simulink model "PMSMSystem"  (R2025a)
settings: Solver=ode45  StartTime=0.0  StopTime=0.2  FixedStep=40e-6  RelTol=1e-3
PreLoadFcn:
  | pmsmfoc_data
StartFcn:
  | clear executionProfile
StopFcn:
  | try
  |   AddExecutionProfileToDataInspector();
  | end
undefined symbols (not defined in the file): ctrlConst, DiscIntNeverNeededParam, EnumCommandType, pmsm, sensors
libraries: fl_lib x13, nesl_utility x11, ee_lib x6, fl_ps_legacy_lib x2, simulink x2, eeTransforms x1, SignalEditorBlockLib x1
Description:
  | Field-Oriented Control of Permanent Magnet Synchronous Machine
  | 
  | Demonstrates a Field-Oriented Control algorithm with Space Vector Modulation for a Permanent Magnet Synchronous Machine (PMSM).
  | The test bench can be used to evaluate the system performance. Examples include turning the motor on, searching for a valid rotor position,
  | transitioning to closed loop operation, and changing speed and torque during closed loop control.
  | The Embedded Processor subsystem contains the controller algorithm (which supports C code generation) as well as simulation models of peripherals.
settings Model: Creator=The MathWorks, Inc.  LastModifiedBy=anubhasinghal
settings SolverCC: AlgebraicLoopSolver=TrustRegion
settings DataIOCC: LimitDataPoints=on  SaveFormat=Array  SaveOutput=off  SaveTime=off
settings OptimizationCC: DefaultParameterBehavior=Inlined  UseFloatMulNetSlope=on  InlineInvariantSignals=on  ReuseModelBlockBuffer=off  EnhancedBackFolding=on  StrengthReduction=on  PassReuseOutputArgsAs=Individual arguments  ExpressionDepthLimit=2147483647.0  ZeroExternalMemoryAtStartup=off  EfficientFloat2IntCast=on  LifeSpan=1  EfficientTunableParamExpr=on
settings DebuggingCC: AlgebraicLoopMsg=error  MergeDetectMultiDrivingBlocksExec=none  SingleTaskRateTransMsg=error  IntegerOverflowMsg=none  ParameterPrecisionLossMsg=none  FcnCallInpInsideContextMsg=warning  UniqueDataStoreMsg=error  AssertControl=DisableAll  AllowSymbolicDim=off  StateNameClashWarn=warning  SubsystemReferenceDiagnosticForUnitTest=warning  SFUnexpectedBacktrackingDiag=warning  SFNoUnconditionalDefaultTransitionDiag=warning  SFExecutionAtInitializationDiag=none  IntegerSaturationMsg=none  ArithmeticOperatorsInVariantConditions=warning
settings ModelReferenceCC: EnableRefExpFcnMdlSchedulingChecks=on  ModelReferenceNumInstancesAllowed=Single  PropagateSignalLabelsOutOfModel=off
settings SFSimCC: SimUseLocalCustomCode=off  MATLABDynamicMemAlloc=off
settings RTWCC: SystemTargetFile=ert.tlc  GenerateMakefile=off  TemplateMakefile=ec_target.tmf  GenerateReport=on  RTWVerbose=off  RTWUseLocalCustomCode=off  IncludeHyperlinkInReport=on  PortableWordSizes=on  CodeExecutionProfiling=on  CodeProfilingSaveOptions=AllData  CodeProfilingInstrumentation=detailed  GenerateTraceInfo=on  GenerateTraceReport=on  GenerateTraceReportSl=on  GenerateTraceReportSf=on  GenerateTraceReportEml=on  GPUComputeCapability=3.5  Description=Embedded Coder
settings CodeAppCC: IgnoreCustomStorageClasses=off  IgnoreTestpoints=on  MaxIdLength=64.0  MATLABFcnDesc=on  CustomSymbolStrGlobalVar=$N$M  CustomSymbolStrType=$N$M  CustomSymbolStrFcn=$N$M$F  CustomSymbolStrFcnArg=$I$N$M  CustomSymbolStrBlkIO=$N$M  CustomSymbolStrMacro=$N$M  StateflowObjectComments=on  MATLABSourceComments=on  InternalIdentifier=Classic
settings ERTTargetCC: ExtModeTransport=0.0  ExtModeStaticAlloc=off  ExtModeMexFile=ext_comm  ExtModeIntrfLevel=Level1  ERTCustomFileTemplate=example_file_process.tlc  ERTFilePackagingFormat=Compact  ConvertIfToSwitch=off  SuppressUnreachableDefaultCases=off  DynamicArrayContainerType=coder::array  MultiwordLength=2048.0  SuppressErrorStatus=on  SupportAbsoluteTime=off  SubcomponentCodeInterfacePackaging=Nonreusable function  SupportNonFinite=off  RemoveResetFunc=off  ParenthesesLevel=Maximum
settings ConfigComp: CovMetricSettings=dcmtrzow  CovHTMLOptions=-aTS=1 -bRG=1 -bTC=1 -hTR=0 -nFC=0 -scm=1 -bcm=1 -xEv=0  CovSaveCumulativeToWorkspaceVar=on  CovSaveSingleToWorkspaceVar=on  CovExternalEMLEnable=off  CovSFcnEnable=off
settings SimscapeCC: SimscapeNormalizeSystem=off

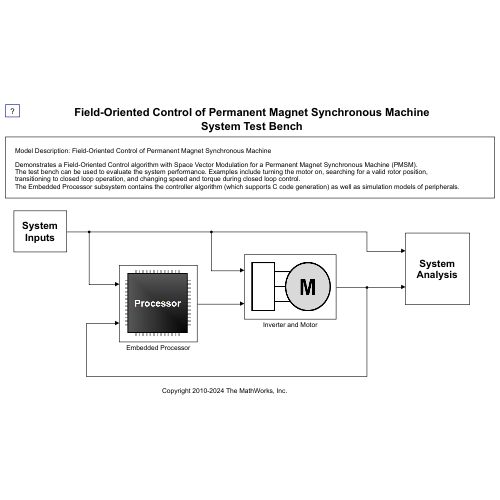
[thumbnail: Simulink's stored preview of the top-level diagram]
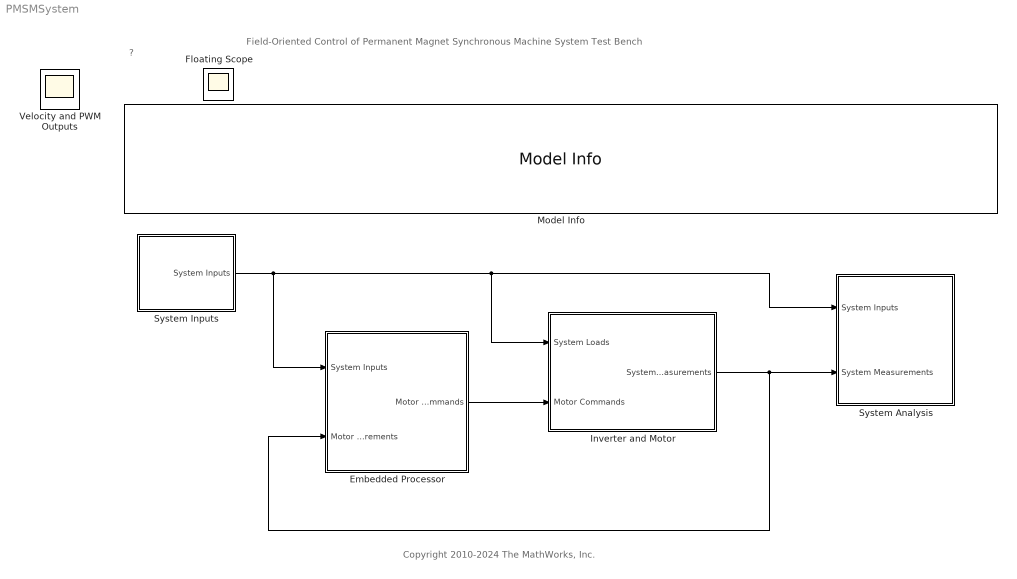
== system PMSMSystem ==
  note: Field-Oriented Control of Permanent Magnet Synchronous Machine
      | System Test Bench
  note: Copyright 2010-2024 The MathWorks, Inc.
  note: ?
  Embedded Processor : Subsystem
      mask Display:
      | if exist('rtwdemo_pmsmfoc_processor.png', 'file')
      |     image('rtwdemo_pmsmfoc_processor.png');
      | end
  Inverter and Motor : Subsystem  Description=""
      mask Display:
      | if exist('rtwdemo_pmsmfoc_motor.png', 'file')
      |     image('rtwdemo_pmsmfoc_motor.png')
      | end
  Model Info : simulink/Model-Wide Utilities/Model Info  Frame=on  DisplayStringWithTags=Model Description: %<Description>  HorizontalTextAlignment=Left  LeftAlignmentValue=0.02
  System Analysis : Subsystem  Description=|
      | System Analysis for Speed Control Design
      | 
      | Analyize and plot signals used to analyize performance of
      | speed  control designs
      mask Display: fprintf('System\nAnalysis')
  System Inputs : Subsystem  Description=""
      mask Display: fprintf('System\nInputs')
  Floating Scope : Scope
  Velocity and PWM Outputs : Scope
      settings: TimeSpan=0.14  ActiveDisplayYMinimum=-500  ActiveDisplayYMaximum=4000  DataLoggingMaxPoints=7500  DataLoggingVariableName=ScopeData4  DataLoggingSaveFormat=Array
  wires:
  Embedded Processor/1(Motor Commands) -> Inverter and Motor/2(Motor Commands)
  Inverter and Motor/1(System Measurements) -> System Analysis/2(System Measurements), Embedded Processor/2(Motor Measurements)
  System Inputs/1(System Inputs) -> System Analysis/1(System Inputs), Inverter and Motor/1(System Loads), Embedded Processor/1(System Inputs)

== system PMSMSystem/Embedded Processor ==
  note: Models hardware on the embedded processor, including
      | the controller algorithm software specification and peripherals.
  note: Embedded Processor
  System Inputs : Inport
  Motor Measurements : Inport  Port=2
  Command Channel : Subsystem  Description=""
      mask Display: fprintf('Command\nChannel')
  Controller Algorithm Software Specification : ModelReference  ModelNameDialog=PMSMController  SimulationMode=Normal  ModelReferenceVersion=11.1
  Driver Peripherals : Subsystem  Description=""
      mask Display: fprintf('Drivers\nPeripherals')
  Sensor Peripherals : Subsystem  Description=|
      | Elaborate Sensor Models
      | 
      | ADC and QEP and Encoder Models
      mask Display: fprintf('Sensor\nPeripherals')
  Motor Commands : Outport  VectorParamsAs1DForOutWhenUnconnected=off
  wires:
  System Inputs/1 -> Command Channel/1(System Inputs)
  Motor Measurements/1 -> Sensor Peripherals/1(System Measurements)
  Driver Peripherals/1(PWM Duty Cycle) -> Motor Commands/1
  Command Channel/1(motor_on) -> Controller Algorithm Software Specification/1  "motor_on"
  Sensor Peripherals/1(Sensors) -> Controller Algorithm Software Specification/4  "sensors"
  Controller Algorithm Software Specification/1 -> Driver Peripherals/1(pwm_compare)  "pwm_compare"
  Command Channel/2(command_type) -> Controller Algorithm Software Specification/2  "command_type"
  Command Channel/3(command_value) -> Controller Algorithm Software Specification/3  "command_value"
  Controller Algorithm Software Specification/2 -> Driver Peripherals/2(error)  "error"

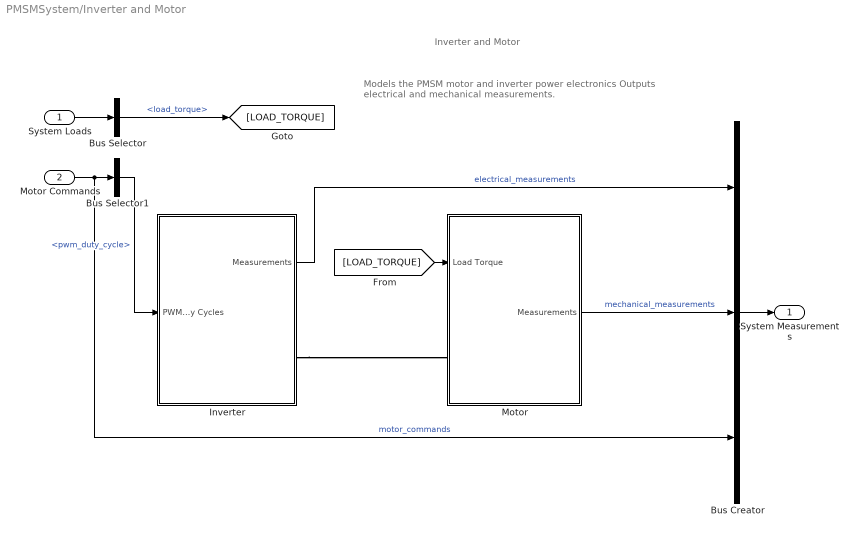
== system PMSMSystem/Inverter and Motor ==
  note: Models the PMSM motor and inverter power electronics
      | Outputs electrical and mechanical measurements.
  note: Inverter and Motor
  System Loads : Inport
  Motor Commands : Inport  Port=2
  Bus Creator : BusCreator  Inputs=3
  Bus Selector : BusSelector  OutputSignals=load_torque
  Bus Selector1 : BusSelector  OutputSignals=pwm_duty_cycle
  Inverter : Subsystem
  Motor : Subsystem
  System Measurements : Outport  VectorParamsAs1DForOutWhenUnconnected=off
  wires:
  Inverter/1(Measurements) -> Bus Creator/1  "electrical_measurements"
  Bus Creator/1 -> System Measurements/1
  Motor/1(Measurements) -> Bus Creator/2  "mechanical_measurements"
  System Loads/1 -> Bus Selector/1
  Motor Commands/1 -> Bus Selector1/1, Bus Creator/3  "motor_commands"
  Bus Selector/1 -> [LOAD_TORQUE]  "<load_torque>"
  Bus Selector1/1 -> Inverter/1(PWM Duty Cycles)  "<pwm_duty_cycle>"
  [LOAD_TORQUE] -> Motor/1("Load Torque ")
  connections:
  Inverter/RConn1 -- Motor/LConn1

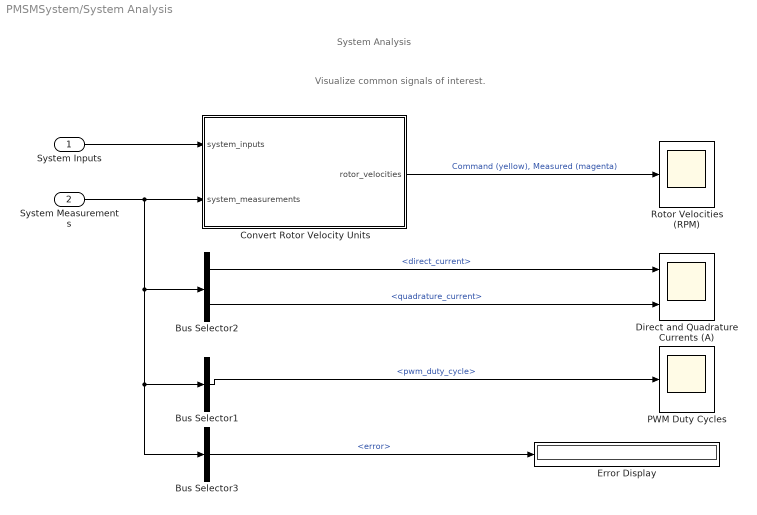
== system PMSMSystem/System Analysis ==
  note: System Analysis
  note: Visualize common signals of interest.
  System Inputs : Inport
  System Measurements : Inport  Port=2
  Bus Selector1 : BusSelector  OutputSignals=motor_commands.pwm_duty_cycle
  Bus Selector2 : BusSelector  OutputSignals=mechanical_measurements.direct_current,mechanical_measurements.quadrature_current
  Bus Selector3 : BusSelector  OutputSignals=motor_commands.error
  Convert Rotor Velocity Units : Subsystem
  Direct and Quadrature Currents (A) : Scope  NumInputPorts=2
      settings: TimeSpan=0.2  ActiveDisplayYMinimum=-0.05574  ActiveDisplayYMaximum=0.11277  DataLoggingVariableName=ScopeData3
  Error Display : Display
  PWM Duty Cycles : Scope
      settings: TimeSpan=1.4  ActiveDisplayYMinimum=0.38629  ActiveDisplayYMaximum=0.61338  DataLoggingVariableName=ScopeData2
  Rotor Velocities (RPM) : Scope
      settings: TimeSpan=0.2  ActiveDisplayYMinimum=-125.00445  ActiveDisplayYMaximum=1125.00049
  wires:
  System Measurements/1 -> Convert Rotor Velocity Units/2(system_measurements), Bus Selector3/1, Bus Selector1/1, Bus Selector2/1
  System Inputs/1 -> Convert Rotor Velocity Units/1(system_inputs)
  Convert Rotor Velocity Units/1(rotor_velocities) -> Rotor Velocities (RPM)/1  "Command (yellow), Measured (magenta)"
  Bus Selector1/1 -> PWM Duty Cycles/1  "<pwm_duty_cycle>"
  Bus Selector2/1 -> Direct and Quadrature Currents (A)/1  "<direct_current>"
  Bus Selector2/2 -> Direct and Quadrature Currents (A)/2  "<quadrature_current>"
  Bus Selector3/1 -> Error Display/1  "<error>"

== system PMSMSystem/System Inputs ==
  note: System Inputs
  note: Specify groups of tests in Signal Builder. Outputs are combined into a bus
      | to simplify signal routing through the model.
  Bus Creator : BusCreator  Inputs=4
  Command Type : simulink/Sources/Enumerated Constant  OutDataTypeStr=Enum: EnumCommandType  Value=EnumCommandType.Velocity  SampleTime=inf
  Signal Editor Experiments : SignalEditorBlockLib/Signal Editor  FileName=rtwdemo_pmsmfoc_system_Signals.mat  ActiveScenario=No_Load_Velocity_Control  ActiveSignal=Load Torque (oz-in)  IsBus=off  OutputBusObjectStr=Bus: BusObject  SampleTime=1e-5  OutputAfterFinalValue=Holding final value  Unit=inherit  PreserveSignalName=on  ApplySigPropsToAllScenarios=on  ApplySigPropsToAllSignals=off  SignalPropertySource=Dialog parameters
  oz-in to Newton Meters : Gain  Gain=0.0070615518333
      settings: AttributesFormatString=-------------------------\n%<Gain>
  rpm to rad per sec : Gain  Gain=pi/30
      settings: AttributesFormatString=------------------\n%<Gain>
  System Inputs : Outport  VectorParamsAs1DForOutWhenUnconnected=off
  wires:
  Bus Creator/1 -> System Inputs/1
  oz-in to Newton Meters/1 -> Bus Creator/4  "load_torque"
  rpm to rad per sec/1 -> Bus Creator/3  "command"
  Command Type/1 -> Bus Creator/1  "command_type"
  Signal Editor Experiments/1 -> Bus Creator/2  "motor_on"
  ? -> rpm to rad per sec/1  "speed_command_rpm"
  ? -> oz-in to Newton Meters/1  "load_torque_ozin"

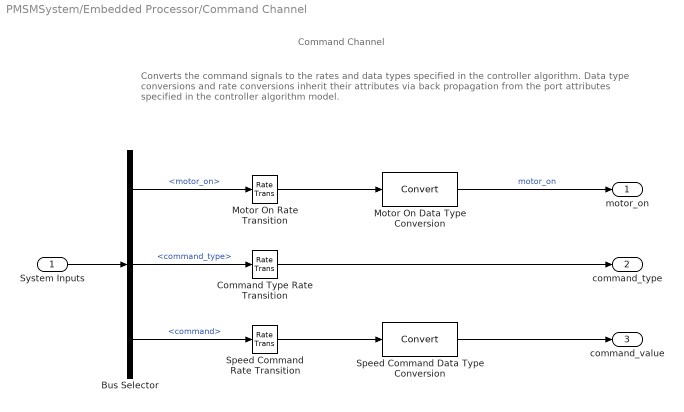
== system PMSMSystem/Embedded Processor/Command Channel ==
  note: Converts the command signals to the rates and data types specified in the controller algorithm.
      | Data type conversions and rate conversions inherit their attributes via back propagation from the
      | port attributes specified in the controller algorithm model.
  note: Command Channel
  System Inputs : Inport
  Bus Selector : BusSelector  OutputSignals=motor_on,command_type,command
  Command Type Rate Transition : RateTransition  Integrity=off  Deterministic=off
  Motor On Data Type Conversion : DataTypeConversion  SaturateOnIntegerOverflow=off  RndMeth=Floor
  Motor On Rate Transition : RateTransition  Integrity=off  Deterministic=off
  Speed Command Data Type Conversion : DataTypeConversion  SaturateOnIntegerOverflow=off  RndMeth=Floor
  Speed Command Rate Transition : RateTransition  Integrity=off  Deterministic=off
  motor_on : Outport  VectorParamsAs1DForOutWhenUnconnected=off
  command_type : Outport  Port=2  VectorParamsAs1DForOutWhenUnconnected=off
  command_value : Outport  Port=3  VectorParamsAs1DForOutWhenUnconnected=off
  wires:
  System Inputs/1 -> Bus Selector/1
  Speed Command Data Type Conversion/1 -> command_value/1
  Bus Selector/1 -> Motor On Rate Transition/1  "<motor_on>"
  Motor On Data Type Conversion/1 -> motor_on/1  "motor_on"
  Motor On Rate Transition/1 -> Motor On Data Type Conversion/1
  Speed Command Rate Transition/1 -> Speed Command Data Type Conversion/1
  Bus Selector/3 -> Speed Command Rate Transition/1  "<command>"
  Bus Selector/2 -> Command Type Rate Transition/1  "<command_type>"
  Command Type Rate Transition/1 -> command_type/1

== system PMSMSystem/Embedded Processor/Driver Peripherals ==
  note: Converts PWM count compare values to a normalized duty cycle.
  note: Driver Peripherals
  pwm_compare : Inport
  error : Inport  Port=2
  Bus Creator : BusCreator  Inputs=2
  Rate Transition : RateTransition  Integrity=off  Deterministic=off  OutPortSampleTime=1e-5
  Units Per PWM Count : Gain  Gain=1 / ctrlConst.PwmCountsPerRevolution  ParamDataTypeStr=double  OutDataTypeStr=double
      settings: AttributesFormatString=------------------------------------------\nGain:\n%<Gain>
  PWM Duty Cycle : Outport  VectorParamsAs1DForOutWhenUnconnected=off
  wires:
  Rate Transition/1 -> Bus Creator/1  "pwm_duty_cycle"
  pwm_compare/1 -> Units Per PWM Count/1
  Units Per PWM Count/1 -> Rate Transition/1
  error/1 -> Bus Creator/2
  Bus Creator/1 -> PWM Duty Cycle/1

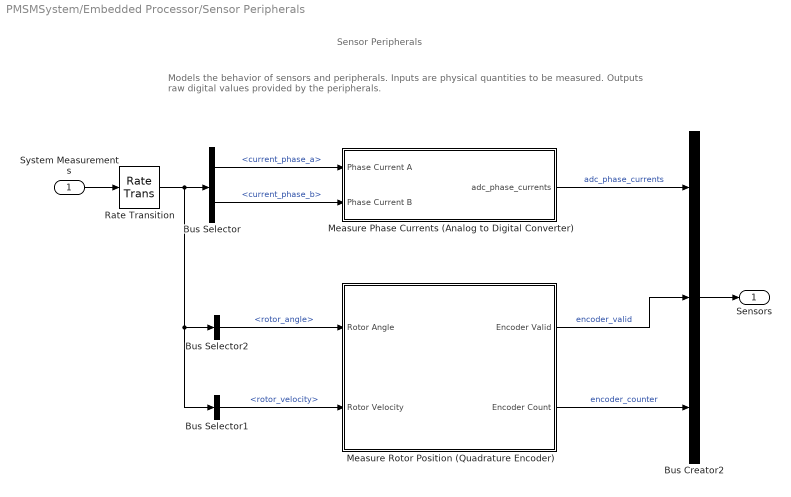
== system PMSMSystem/Embedded Processor/Sensor Peripherals ==
  note: Models the behavior of sensors and peripherals.
      | Inputs are physical quantities to be measured. Outputs raw digital values provided by the peripherals.
  note: Sensor Peripherals
  System Measurements : Inport
  Bus Creator2 : BusCreator  Inputs=3  OutDataTypeStr=Bus: SENSORS_STRUCT
  Bus Selector : BusSelector  OutputSignals=mechanical_measurements.current_phase_a,mechanical_measurements.current_phase_b
  Bus Selector1 : BusSelector  OutputSignals=mechanical_measurements.rotor_velocity
  Bus Selector2 : BusSelector  OutputSignals=mechanical_measurements.rotor_angle
  Measure Phase Currents (Analog to Digital Converter) : Subsystem
  Measure Rotor Position (Quadrature Encoder) : Subsystem
  Rate Transition : RateTransition  OutPortSampleTime=40e-6
  Sensors : Outport  VectorParamsAs1DForOutWhenUnconnected=off
  wires:
  Measure Phase Currents (Analog to Digital Converter)/1(adc_phase_currents) -> Bus Creator2/1  "adc_phase_currents"
  Bus Selector2/1 -> Measure Rotor Position (Quadrature Encoder)/1(Rotor Angle)  "<rotor_angle>"
  Bus Selector1/1 -> Measure Rotor Position (Quadrature Encoder)/2(Rotor Velocity)  "<rotor_velocity>"
  System Measurements/1 -> Rate Transition/1
  Bus Creator2/1 -> Sensors/1
  Measure Rotor Position (Quadrature Encoder)/1(Encoder Valid) -> Bus Creator2/2  "encoder_valid"
  Measure Rotor Position (Quadrature Encoder)/2(Encoder Count) -> Bus Creator2/3  "encoder_counter"
  Bus Selector/1 -> Measure Phase Currents (Analog to Digital Converter)/1(Phase Current A)  "<current_phase_a>"
  Bus Selector/2 -> Measure Phase Currents (Analog to Digital Converter)/2(Phase Current B)  "<current_phase_b>"
  Rate Transition/1 -> Bus Selector1/1, Bus Selector2/1, Bus Selector/1

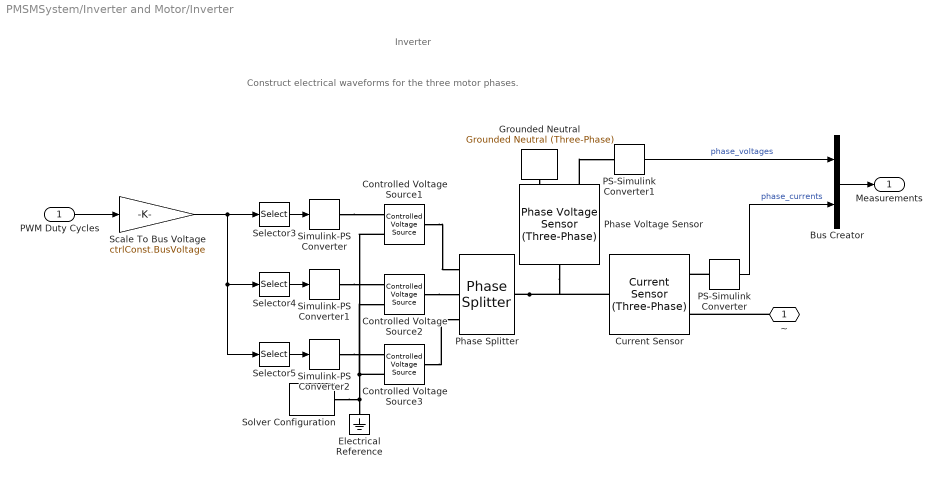
== system PMSMSystem/Inverter and Motor/Inverter ==
  note: Construct electrical waveforms for the three motor phases.
  note: Inverter
  PWM Duty Cycles : Inport
  Bus Creator : BusCreator  Inputs=2
  Controlled Voltage Source1 : fl_lib/Electrical/Electrical Sources/Controlled Voltage Source
  Controlled Voltage Source2 : fl_lib/Electrical/Electrical Sources/Controlled Voltage Source
  Controlled Voltage Source3 : fl_lib/Electrical/Electrical Sources/Controlled Voltage Source
  Current Sensor : ee_lib/Sensors & Transducers/Current Sensor (Three-Phase)
  Electrical Reference : fl_lib/Electrical/Electrical Elements/Electrical Reference
  Grounded Neutral : ee_lib/Connectors & References/Grounded Neutral (Three-Phase)
  PS-Simulink Converter : nesl_utility/PS-Simulink Converter  PhysicalDomain=network_engine_domain  SubClassName=ps_output  LeftPortType=input  RightPortType=output  PseudoPeriodic=off  Frequencies=[]  VectorFormat=1-D array  Unit=A  AffineConversion=off
  PS-Simulink Converter1 : nesl_utility/PS-Simulink Converter  PhysicalDomain=network_engine_domain  SubClassName=ps_output  LeftPortType=input  RightPortType=output  PseudoPeriodic=off  Frequencies=[]  VectorFormat=1-D array  Unit=V  AffineConversion=off
  Phase Splitter : ee_lib/Connectors & References/Phase Splitter
  Phase Voltage Sensor : ee_lib/Sensors & Transducers/Phase Voltage Sensor (Three-Phase)
  Scale To Bus Voltage : Gain  Gain=ctrlConst.BusVoltage  ParamDataTypeStr=double  OutDataTypeStr=double
      settings: AttributesFormatString=------------------------------\nGain:\n%<Gain>
  Selector3 : Selector  InputPortWidth=3  IndexOptions=Index vector (dialog)  Indices=[1]  OutputSizes=1
  Selector4 : Selector  InputPortWidth=3  IndexOptions=Index vector (dialog)  Indices=2  OutputSizes=1
  Selector5 : Selector  InputPortWidth=3  IndexOptions=Index vector (dialog)  Indices=3  OutputSizes=1
  Simulink-PS Converter : nesl_utility/Simulink-PS Converter  PhysicalDomain=network_engine_domain  SubClassName=ps_input  LeftPortType=input  RightPortType=output  PseudoPeriodic=off  Frequencies=[]  NoiseDistribution=none  NoiseParameters=[]  Unit=1  AffineConversion=off  FilteringAndDerivatives=provide  SimscapeFilterOrder=1  InputFilterTimeConstant=0.001  UdotUserProvided=0
  Simulink-PS Converter1 : nesl_utility/Simulink-PS Converter  PhysicalDomain=network_engine_domain  SubClassName=ps_input  LeftPortType=input  RightPortType=output  PseudoPeriodic=off  Frequencies=[]  NoiseDistribution=none  NoiseParameters=[]  Unit=1  AffineConversion=off  FilteringAndDerivatives=provide  SimscapeFilterOrder=1  InputFilterTimeConstant=0.001  UdotUserProvided=0
  Simulink-PS Converter2 : nesl_utility/Simulink-PS Converter  PhysicalDomain=network_engine_domain  SubClassName=ps_input  LeftPortType=input  RightPortType=output  PseudoPeriodic=off  Frequencies=[]  NoiseDistribution=none  NoiseParameters=[]  Unit=1  AffineConversion=off  FilteringAndDerivatives=provide  SimscapeFilterOrder=1  InputFilterTimeConstant=0.001  UdotUserProvided=0
  Solver Configuration : nesl_utility/Solver Configuration  PhysicalDomain=network_engine_domain  SubClassName=solver  LeftPortType=input  RightPortType=generic  Tones=[]  Harmonics=[]  SimulateNoise=off  Profile=off  UseLocalSampling=off  EnableSwitchedLinearOptims=on  FrequencyDomain=off  UseCCode=off  RelTol=0.001  AbsTol=1e-06  MinStep=1e-09  ToWorkspace=off  RevertToSquareIcSolve=off  NumHomotopyIterations=100  PhasorMode=off  PhasorModeNumHarmonics=1  ConsistencySolver=NEWTON_FTOL  IndexReductionMethod=DerivativeReplacement  DoDC=off  ResidualTolerance=1e-09  ConsistencyTolSource=GLOBAL  ConsistencyAbsTol=0.001  ConsistencyRelTol=0.001  ConsistencyTolFactor=0.001  UseLocalSolver=on  LocalSolverChoice=NE_BACKWARD_EULER_ADVANCER  ResolveIndetEquations=on  FunctionEvalNumThread=1  LocalSolverSampleTime=1e-5  DoFixedCost=on  MaxNonlinIter=3  MaxModeIter=2  ComputeImpulses=off  ImpulseIterations=2  LinearAlgebra=Sparse  LinearAlgebraNumThread=0  EquationFormulation=NE_TIME_EF  DelaysMemoryBudget=1024  AutomaticFiltering=on  FilteringTimeConstant=0.001  PartitionStorageMethod=AS_NEEDED  PartitionMemoryBudget=1024  PartitionMethod=FAST  MultibodyUseLocalSolver=off  MultibodyLocalSolverChoice=ODE1  MultibodyLocalSolverSampleTime=0.001
  ~ : PMIOPort  Side=Right
  Measurements : Outport  VectorParamsAs1DForOutWhenUnconnected=off
  wires:
  PWM Duty Cycles/1 -> Scale To Bus Voltage/1
  PS-Simulink Converter/1 -> Bus Creator/2  "phase_currents"
  PS-Simulink Converter1/1 -> Bus Creator/1  "phase_voltages"
  Bus Creator/1 -> Measurements/1
  Selector3/1 -> Simulink-PS Converter/1
  Selector4/1 -> Simulink-PS Converter1/1
  Selector5/1 -> Simulink-PS Converter2/1
  Scale To Bus Voltage/1 -> Selector4/1, Selector5/1, Selector3/1
  connections:
  Electrical Reference/LConn1 -- Controlled Voltage Source1/RConn2 -- Controlled Voltage Source2/RConn2 -- Controlled Voltage Source3/RConn2 -- Solver Configuration/RConn1
  Phase Splitter/LConn1 -- Current Sensor/LConn1 -- Phase Voltage Sensor/LConn1
  Grounded Neutral/LConn1 -- Phase Voltage Sensor/RConn2
  Controlled Voltage Source3/LConn1 -- Phase Splitter/RConn3
  PS-Simulink Converter/LConn1 -- Current Sensor/RConn1
  ~/RConn1 -- Current Sensor/RConn2
  Controlled Voltage Source2/LConn1 -- Phase Splitter/RConn2
  Controlled Voltage Source1/LConn1 -- Phase Splitter/RConn1
  Simulink-PS Converter2/RConn1 -- Controlled Voltage Source3/RConn1
  Phase Voltage Sensor/RConn1 -- PS-Simulink Converter1/LConn1
  Simulink-PS Converter1/RConn1 -- Controlled Voltage Source2/RConn1
  Simulink-PS Converter/RConn1 -- Controlled Voltage Source1/RConn1

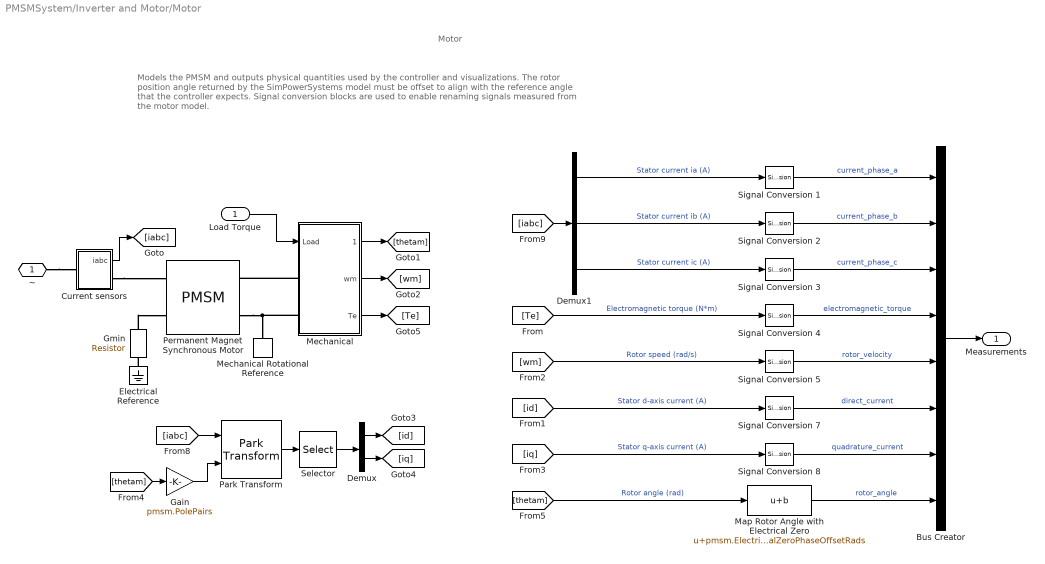
== system PMSMSystem/Inverter and Motor/Motor ==
  note: Motor
  note: Models the PMSM and outputs physical quantities used by the controller and visualizations.
      | The rotor position angle returned by the SimPowerSystems model must be offset to align with the reference angle that the controller expects.
      | Signal conversion blocks are used to enable renaming signals measured from the motor model.
  "Load Torque " : Inport
  Bus Creator : BusCreator  Inputs=8
  Current sensors : Subsystem
  Demux : Demux  Outputs=2
  Demux1 : Demux  Outputs=3
  Electrical Reference : fl_lib/Electrical/Electrical Elements/Electrical Reference
  Gain : Gain  Gain=pmsm.PolePairs
  Gmin : fl_lib/Electrical/Electrical Elements/Resistor  R=1e9 Ohm  i_specify=off  i_priority=None  i=0 A  i_nominal_specify=off  i_nominal_value=1  i_nominal_unit=A  v_specify=off  v_priority=None  v=0 V  v_nominal_specify=off  v_nominal_value=1  v_nominal_unit=V
  Map Rotor Angle with Electrical Zero : Bias  Bias=pmsm.ElectricalZeroPhaseOffsetRads  SaturateOnIntegerOverflow=off
      settings: AttributesFormatString=----------------------------------------\n%<Bias>
  Mechanical : Subsystem
  Mechanical Rotational Reference : fl_lib/Mechanical/Rotational Elements/Mechanical Rotational Reference
  Park Transform : eeTransforms/Park Transform  AxisAlignment=Q-axis  PowerInvariant=off
  Permanent Magnet Synchronous Motor : ee_lib/Electromechanical/Permanent Magnet/PMSM  port_option=ee.enum.threePhasePort.composite  winding_type=ee.enum.statorconnection.wye  machine_param=ee.enum.pmsm.parameterization.constant  nPolePairs=pmsm.PolePairs  pmflux_param=1  pm_flux_linkage=pmsm.TorqueConstant/(1.5*pmsm.PolePairs) Wb  torque_constant=0.18 N*m/A  back_emf_constant=0.18 V/(rad/s)  stator_param=1  Ld=pmsm.InductanceLd H  Lq=pmsm.InductanceLq H  idVec=[-200, 0, 200] A  iqVec=[-200, 0, 200] A  LdMatrix=0.0002 * ones(3, 3) H  LqMatrix=0.0002 * ones(3, 3) H  PmMatrix=0.1 * ones(3, 3) Wb  ktMatrix=0.18 * ones(3, 3) N*m/A  keMatrix=0.18 * ones(3, 3) V/(rad/s)  L0=0.00016 H  Ls=0.0002 H  Lm=-0.00002 H  Ms=0.00002 H  Rs=pmsm.StatorPhaseResistance Ohm  zero_sequence=ee.enum.park.zerosequence.include  axes_param=1  loss_param=ee.enum.ironloss.none  losses_oc=[0, 0, 0] W  losses_sc=[0, 0, 0] W  f_losses=60 Hz  Isc_losses=95 A  J=0 kg*m^2  lam=0 N*m/(rad/s)  i_d_specify=off  i_d_priority=None  i_d=0 A  i_d_nominal_specify=off  i_d_nominal_value=1  i_d_nominal_unit=A  i_q_specify=off  i_q_priority=None  i_q=0 A  i_q_nominal_specify=off  i_q_nominal_value=1  i_q_nominal_unit=A  torque_specify=off  torque_priority=None  torque=0 N*m  torque_nominal_specify=off  torque_nominal_value=1  torque_nominal_unit=N*m  angular_velocity_specify=off  angular_velocity_priority=High  angular_velocity=0 rpm  angular_velocity_nominal_specify=off  angular_velocity_nominal_value=1  angular_velocity_nominal_unit=rpm  angular_position_specify=on  angular_position_priority=High  angular_position=pmsm.ThetaInitDegrees deg  angular_position_nominal_specify=off  angular_position_nominal_value=1  angular_position_nominal_unit=deg  alpha=3.93e-3 1/K  alpha_flux=-0.001 1/K  Tmeas=298.15 K  stator_thermal_mass=100 J/K  rotor_thermal_mass=200 J/K  Rm_percent_rotor=90  Rd_percent_rotor=30  temperatureA_specify=off  temperatureA_priority=High  temperatureA=25 degC  temperatureA_nominal_specify=off  temperatureA_nominal_value=1  temperatureA_nominal_unit=degC  temperatureB_specify=off  temperatureB_priority=High  temperatureB=25 degC  temperatureB_nominal_specify=off  temperatureB_nominal_value=1  temperatureB_nominal_unit=degC  temperatureC_specify=off  temperatureC_priority=High  temperatureC=25 degC  temperatureC_nominal_specify=off  temperatureC_nominal_value=1  temperatureC_nominal_unit=degC  temperatureR_specify=off  temperatureR_priority=High  temperatureR=25 degC  temperatureR_nominal_specify=off  temperatureR_nominal_value=1  temperatureR_nominal_unit=degC
      settings: InternalSimscapePortConfiguration="{\"Bottom\":[],\"Left\":[{\"id\":\"N\",\"label\":\"~\",\"type\":\"foundation.electrical.three_phase\"},{\"id\":\"n\",\"label\":\"n\",\"type\":\"foundation.electrical.electrical\"}],\"Right\":[{\"id\":\"R\",\"label\":\"R\",\"type\":\"foundation.mechanical.rotational.rotational\"},{\"id\":\"C\",\"label\":\"C\",\"type\":\"foundation.mechanical.rotational.rotational\"}],\"Top\":[]}"
  Selector : Selector  InputPortWidth=3  IndexOptions=Index vector (dialog)  Indices=[1 2]  OutputSizes=1
  Signal Conversion {1..5,7..8} (7 alike) : SignalConversion  ConversionOutput=Contiguous copy  OverrideOpt=off
  ~ : PMIOPort  Side=Left
  Measurements : Outport  VectorParamsAs1DForOutWhenUnconnected=off
  wires:
  Demux1/1 -> Signal Conversion 1/1  "Stator current ia (A)"
  Demux1/2 -> Signal Conversion 2/1  "Stator current ib (A)"
  Demux1/3 -> Signal Conversion 3/1  "Stator current ic (A)"
  [wm] -> Signal Conversion 5/1  "Rotor speed (rad/s)"
  [Te] -> Signal Conversion 4/1  "Electromagnetic torque (N*m)"
  Bus Creator/1 -> Measurements/1
  Signal Conversion 1/1 -> Bus Creator/1  "current_phase_a"
  Signal Conversion 2/1 -> Bus Creator/2  "current_phase_b"
  Signal Conversion 3/1 -> Bus Creator/3  "current_phase_c"
  Signal Conversion 4/1 -> Bus Creator/4  "electromagnetic_torque"
  Signal Conversion 5/1 -> Bus Creator/5  "rotor_velocity"
  [thetam] -> Map Rotor Angle with Electrical Zero/1  "Rotor angle (rad)"
  Signal Conversion 7/1 -> Bus Creator/6  "direct_current"
  Signal Conversion 8/1 -> Bus Creator/7  "quadrature_current"
  Map Rotor Angle with Electrical Zero/1 -> Bus Creator/8  "rotor_angle"
  [id] -> Signal Conversion 7/1  "Stator d-axis current (A)"
  [iq] -> Signal Conversion 8/1  "Stator q-axis current (A)"
  [iabc] -> Park Transform/1
  [thetam] -> Gain/1
  Gain/1 -> Park Transform/2
  Park Transform/1 -> Selector/1
  Selector/1 -> Demux/1
  Demux/1 -> [id]
  Demux/2 -> [iq]
  Current sensors/1(iabc) -> [iabc]
  [iabc] -> Demux1/1
  "Load Torque "/1 -> Mechanical/1(Load)
  Mechanical/1(Thetam) -> [thetam]
  Mechanical/2(wm) -> [wm]
  Mechanical/3(Te) -> [Te]
  connections:
  Gmin/LConn1 -- Permanent Magnet Synchronous Motor/LConn2
  Electrical Reference/LConn1 -- Gmin/RConn1
  Permanent Magnet Synchronous Motor/RConn2 -- Mechanical/LConn2 -- Mechanical Rotational Reference/LConn1
  Current sensors/RConn1 -- Permanent Magnet Synchronous Motor/LConn1
  ~/RConn1 -- Current sensors/LConn1
  Mechanical/LConn1 -- Permanent Magnet Synchronous Motor/RConn1

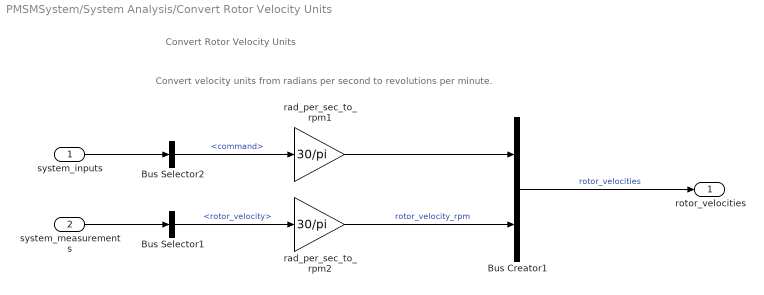
== system PMSMSystem/System Analysis/Convert Rotor Velocity Units ==
  note: Convert Rotor Velocity Units
  note: Convert velocity units from radians per second to revolutions per minute.
  system_inputs : Inport
  system_measurements : Inport  Port=2
  Bus Creator1 : BusCreator  Inputs=2
  Bus Selector1 : BusSelector  OutputSignals=mechanical_measurements.rotor_velocity
  Bus Selector2 : BusSelector  OutputSignals=command
  rad_per_sec_to_rpm1 : Gain  Gain=30/pi
  rad_per_sec_to_rpm2 : Gain  Gain=30/pi
  rotor_velocities : Outport  VectorParamsAs1DForOutWhenUnconnected=off
  wires:
  Bus Selector2/1 -> rad_per_sec_to_rpm1/1  "<command>"
  Bus Selector1/1 -> rad_per_sec_to_rpm2/1  "<rotor_velocity>"
  Bus Creator1/1 -> rotor_velocities/1  "rotor_velocities"
  system_inputs/1 -> Bus Selector2/1
  system_measurements/1 -> Bus Selector1/1
  rad_per_sec_to_rpm1/1 -> Bus Creator1/1
  rad_per_sec_to_rpm2/1 -> Bus Creator1/2  "rotor_velocity_rpm"

== system PMSMSystem/Embedded Processor/Sensor Peripherals/Measure Phase Currents (Analog to Digital Converter) ==
  note: Models the behavior of the current sensor and analog to digital voltage conversion.
  note: Measure Phase Currents
      | (Analog to Digital Converter)
  Phase Current A : Inport
  Phase Current B : Inport  Port=2
  Current Sensor : Subsystem
  Driver Noise : Subsystem
      mask init:
      | if evalin('base','sensors.ADC.NoiseEnable')
      |     enable = 'Enabled';
      | else
      |     enable = 'Disabled';
      | end
      mask Display: fprintf(['ADC Driver Noise\n(' enable ')'])
  Vector Concatenate : Concatenate
  adc_phase_currents : Outport  PortDimensions=[2,1]  VectorParamsAs1DForOutWhenUnconnected=off
  wires:
  Current Sensor/1(Driver Units) -> Driver Noise/1(In)
  Vector Concatenate/1 -> Current Sensor/1(Phase Currents)
  Driver Noise/1(Out) -> adc_phase_currents/1
  Phase Current A/1 -> Vector Concatenate/1
  Phase Current B/1 -> Vector Concatenate/2

== system PMSMSystem/Embedded Processor/Sensor Peripherals/Measure Rotor Position (Quadrature Encoder) ==
  note: Models the behavior of a relative quadrature encoder. The rotor angle and rotor velocity inputs are "ideal" measurements from the motor model.
      | When the motor begins spinning the counter is initialized to some value (assume 0).
      | Once an index pulse is received, the count value is reset to a value corresponding to a valid rotor position.
      | Hence, after the first index pulse is received, the count returned by the peripheral represents the absolute position of the encoder.
  note: Measure Rotor Position
      | (Quadrature Encoder)
  Rotor Angle : Inport
  Rotor Velocity : Inport  Port=2
  Create Index Pulse : MATLAB Function  TreatAsAtomicUnit=on
  Encoder Count (During Startup) : Subsystem
  Encoder Count (Valid After First Index Pulse) : Subsystem
  Select Encoder Count : Subsystem
  Encoder Valid : Outport  VectorParamsAs1DForOutWhenUnconnected=off
  Encoder Count : Outport  Port=2  VectorParamsAs1DForOutWhenUnconnected=off
  wires:
  Select Encoder Count/1(Count) -> Encoder Count/1
  Create Index Pulse/1(indexPulse) -> Select Encoder Count/2(Index)
  Encoder Count (Valid After First Index Pulse)/1(Encoder Count) -> Select Encoder Count/3(Absolute), Create Index Pulse/1(currentCount)
  Encoder Count (During Startup)/1(Encoder Count) -> Select Encoder Count/1(Startup)
  Rotor Velocity/1 -> Encoder Count (During Startup)/1(Rotor Velocity)
  Rotor Angle/1 -> Encoder Count (Valid After First Index Pulse)/1(Rotor Angle)
  Select Encoder Count/2(Valid) -> Encoder Valid/1

== system PMSMSystem/Inverter and Motor/Motor/Current sensors ==
  Current Sensor : ee_lib/Sensors & Transducers/Current Sensor (Three-Phase)
  PS-Simulink Converter : nesl_utility/PS-Simulink Converter  PhysicalDomain=network_engine_domain  SubClassName=ps_output  LeftPortType=input  RightPortType=output  PseudoPeriodic=off  Frequencies=[]  VectorFormat=1-D array  Unit=A  AffineConversion=off
  Unit Delay : UnitDelay  SampleTime=-1  HasFrameUpgradeWarning=on
  ~1 : PMIOPort  Side=Left
  ~2 : PMIOPort  Port=2  Side=Right
  iabc : Outport  VectorParamsAs1DForOutWhenUnconnected=off
  wires:
  PS-Simulink Converter/1 -> Unit Delay/1
  Unit Delay/1 -> iabc/1
  connections:
  PS-Simulink Converter/LConn1 -- Current Sensor/RConn1
  Current Sensor/LConn1 -- ~1/RConn1
  Current Sensor/RConn2 -- ~2/RConn1

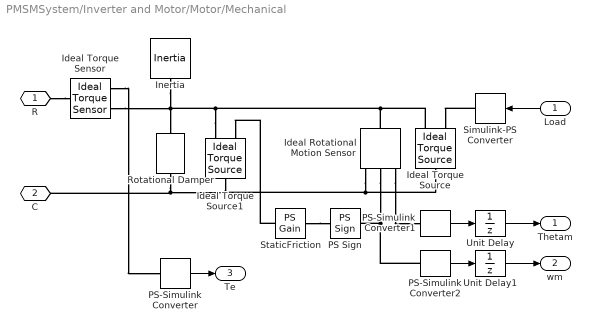
== system PMSMSystem/Inverter and Motor/Motor/Mechanical ==
  Load : Inport
  Ideal Rotational Motion Sensor : fl_lib/Mechanical/Mechanical Sensors/Ideal Rotational Motion Sensor  reference=foundation.enum.MeasurementReference.difference  acceleration_port=false  velocity_port=true  position_port=true  wrap_angle=simscape.enum.onoff.off  offset=pmsm.ThetaInitDegrees deg
  Ideal Torque Sensor : fl_lib/Mechanical/Mechanical Sensors/Ideal Torque Sensor
  Ideal Torque Source : fl_lib/Mechanical/Mechanical Sources/Ideal Torque Source
  Ideal Torque Source1 : fl_lib/Mechanical/Mechanical Sources/Ideal Torque Source
  Inertia : fl_lib/Mechanical/Rotational Elements/Inertia  inertia=pmsm.Inertia kg*m^2  num_ports=foundation.enum.numPorts2.one  w_specify=on  w_priority=High  w=0 rad/s  w_nominal_specify=off  w_nominal_value=1  w_nominal_unit=rad/s  t_specify=off  t_priority=High  t=0 N*m  t_nominal_specify=off  t_nominal_value=1  t_nominal_unit=N*m
  PS Sign : fl_ps_legacy_lib/Legacy Physical Signals/Nonlinear Operators/PS Sign
      settings: InternalSimscapePortConfiguration="{\"Bottom\":[],\"Left\":[{\"id\":\"I\",\"label\":\"\",\"type\":\"input\"}],\"Right\":[{\"id\":\"O\",\"label\":\"\",\"type\":\"output\"}],\"Top\":[]}"
  PS-Simulink Converter : nesl_utility/PS-Simulink Converter  PhysicalDomain=network_engine_domain  SubClassName=ps_output  LeftPortType=input  RightPortType=output  PseudoPeriodic=off  Frequencies=[]  VectorFormat=1-D array  Unit=N*m  AffineConversion=off
  PS-Simulink Converter1 : nesl_utility/PS-Simulink Converter  PhysicalDomain=network_engine_domain  SubClassName=ps_output  LeftPortType=input  RightPortType=output  PseudoPeriodic=off  Frequencies=[]  VectorFormat=1-D array  Unit=rad  AffineConversion=off
  PS-Simulink Converter2 : nesl_utility/PS-Simulink Converter  PhysicalDomain=network_engine_domain  SubClassName=ps_output  LeftPortType=input  RightPortType=output  PseudoPeriodic=off  Frequencies=[]  VectorFormat=1-D array  Unit=rad/s  AffineConversion=off
  Rotational Damper : fl_lib/Mechanical/Rotational Elements/Rotational Damper  D=pmsm.ViscousDamping N*m/(rad/s)  w_specify=off  w_priority=None  w=0 rad/s  w_nominal_specify=off  w_nominal_value=1  w_nominal_unit=rad/s  t_specify=off  t_priority=None  t=0 N*m  t_nominal_specify=off  t_nominal_value=1  t_nominal_unit=N*m
  Simulink-PS Converter : nesl_utility/Simulink-PS Converter  PhysicalDomain=network_engine_domain  SubClassName=ps_input  LeftPortType=input  RightPortType=output  PseudoPeriodic=off  Frequencies=[]  NoiseDistribution=none  NoiseParameters=[]  Unit=1  AffineConversion=off  FilteringAndDerivatives=provide  SimscapeFilterOrder=1  InputFilterTimeConstant=0.001  UdotUserProvided=0
  StaticFriction : fl_ps_legacy_lib/Legacy Physical Signals/Functions/PS Gain  gain=pmsm.StaticFriction
  Unit Delay : UnitDelay  InitialCondition=pmsm.ThetaInitDegrees/180*pi  SampleTime=-1  HasFrameUpgradeWarning=on
  Unit Delay1 : UnitDelay  SampleTime=-1  HasFrameUpgradeWarning=on
  R : PMIOPort  Side=Left
  C : PMIOPort  Port=2  Side=Left
  Thetam : Outport  VectorParamsAs1DForOutWhenUnconnected=off
  wm : Outport  Port=2  VectorParamsAs1DForOutWhenUnconnected=off
  Te : Outport  Port=3  VectorParamsAs1DForOutWhenUnconnected=off
  wires:
  Load/1 -> Simulink-PS Converter/1
  PS-Simulink Converter1/1 -> Unit Delay/1
  PS-Simulink Converter2/1 -> Unit Delay1/1
  PS-Simulink Converter/1 -> Te/1
  Unit Delay/1 -> Thetam/1
  Unit Delay1/1 -> wm/1
  connections:
  Simulink-PS Converter/RConn1 -- Ideal Torque Source/RConn1
  StaticFriction/LConn1 -- PS Sign/RConn1
  StaticFriction/RConn1 -- Ideal Torque Source1/RConn1
  Rotational Damper/RConn1 -- C/RConn1 -- Ideal Torque Source/LConn1 -- Ideal Rotational Motion Sensor/RConn1 -- Ideal Torque Source1/LConn1
  Ideal Torque Source1/RConn2 -- Inertia/LConn1 -- Ideal Torque Sensor/RConn1 -- Rotational Damper/LConn1 -- Ideal Rotational Motion Sensor/LConn1 -- Ideal Torque Source/RConn2
  Ideal Rotational Motion Sensor/RConn2 -- PS Sign/LConn1 -- PS-Simulink Converter2/LConn1
  Ideal Rotational Motion Sensor/RConn3 -- PS-Simulink Converter1/LConn1
  R/RConn1 -- Ideal Torque Sensor/LConn1
  Ideal Torque Sensor/RConn2 -- PS-Simulink Converter/LConn1

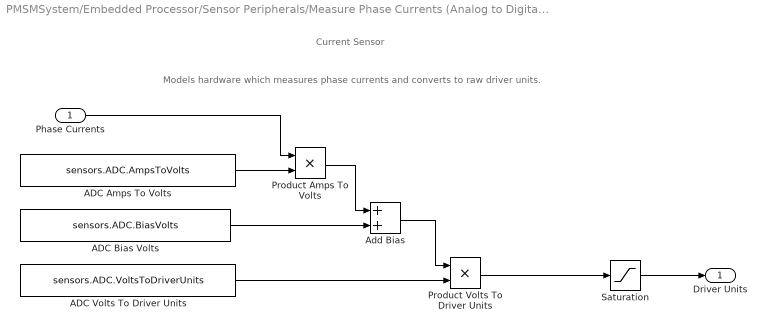
== system PMSMSystem/Embedded Processor/Sensor Peripherals/Measure Phase Currents (Analog to Digital Converter)/Current Sensor ==
  note: Current Sensor
  note: Models hardware which measures phase currents and converts to raw driver units.
  Phase Currents : Inport
  ADC Amps To Volts : Constant  Value=sensors.ADC.AmpsToVolts
  ADC Bias Volts : Constant  Value=sensors.ADC.BiasVolts
  ADC Volts To Driver Units : Constant  Value=sensors.ADC.VoltsToDriverUnits
  Add Bias : Sum
  Product Amps To Volts : Product  RndMeth=Zero
  Product Volts To Driver Units : Product  RndMeth=Zero
  Saturation : Saturate  UpperLimit=sensors.ADC.MaxDriverUnits  LowerLimit=0  OutDataTypeStr=uint16
      settings: AttributesFormatString=----------------------------\nUpper Limit: %<UpperLimit>\nLower Limit: %<LowerLimit>
  Driver Units : Outport  VectorParamsAs1DForOutWhenUnconnected=off
  wires:
  Phase Currents/1 -> Product Amps To Volts/1
  ADC Amps To Volts/1 -> Product Amps To Volts/2
  Product Amps To Volts/1 -> Add Bias/1
  ADC Bias Volts/1 -> Add Bias/2
  Add Bias/1 -> Product Volts To Driver Units/1
  ADC Volts To Driver Units/1 -> Product Volts To Driver Units/2
  Product Volts To Driver Units/1 -> Saturation/1
  Saturation/1 -> Driver Units/1

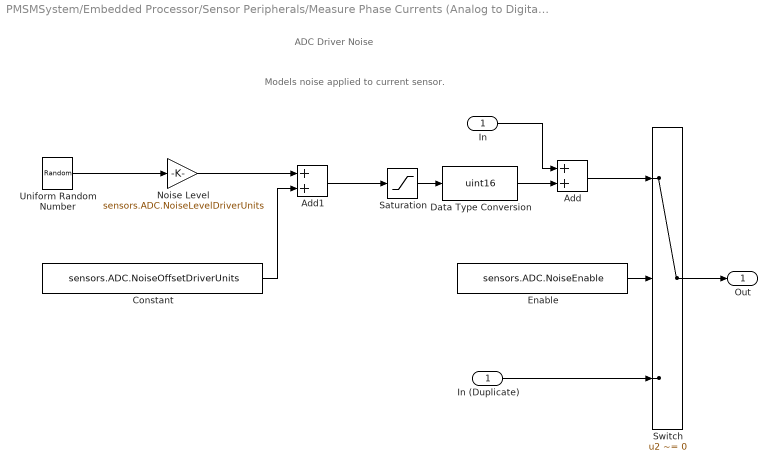
== system PMSMSystem/Embedded Processor/Sensor Peripherals/Measure Phase Currents (Analog to Digital Converter)/Driver Noise ==
  note: ADC Driver Noise
  note: Models noise applied to current sensor.
  In : Inport
  Add : Sum  RndMeth=Convergent  SaturateOnIntegerOverflow=on
  Add1 : Sum  RndMeth=Convergent  SaturateOnIntegerOverflow=on
  Constant : Constant  Value=sensors.ADC.NoiseOffsetDriverUnits
  Data Type Conversion : DataTypeConversion  OutDataTypeStr=uint16  RndMeth=Convergent  SaturateOnIntegerOverflow=off
  Enable : Constant  Value=sensors.ADC.NoiseEnable
  In (Duplicate) : InportShadow
  Noise Level : Gain  Gain=sensors.ADC.NoiseLevelDriverUnits
      settings: AttributesFormatString=------------------------------------\n%<Gain>
  Saturation : Saturate  UpperLimit=sensors.ADC.MaxDriverUnits  LowerLimit=0  OutDataTypeStr=uint16
      settings: AttributesFormatString=----------------------------\nUpper Limit: %<UpperLimit>\nLower Limit: %<LowerLimit>
  Switch : Switch  Criteria=u2 ~= 0  SaturateOnIntegerOverflow=off  InputSameDT=off
  Uniform Random Number : UniformRandomNumber  Minimum=[0 0]  Maximum=[1 1]  SampleTime=ctrlConst.TsHi
  Out : Outport  VectorParamsAs1DForOutWhenUnconnected=off
  wires:
  Switch/1 -> Out/1
  Uniform Random Number/1 -> Noise Level/1
  Noise Level/1 -> Add1/1
  Constant/1 -> Add1/2
  Add1/1 -> Saturation/1
  Saturation/1 -> Data Type Conversion/1
  Add/1 -> Switch/1
  In/1 -> Add/1
  Data Type Conversion/1 -> Add/2
  In (Duplicate)/1 -> Switch/3
  Enable/1 -> Switch/2

== system PMSMSystem/Embedded Processor/Sensor Peripherals/Measure Rotor Position (Quadrature Encoder)/Encoder Count (During Startup) ==
  note: Approximate the count value provided by the encoder peripheral during startup (before reaching the first index pulse).
      | The pulse train generated by the encoder is not modeled.
  note: Encoder Count (During Startup)
  Rotor Velocity : Inport
  Counts per Radian : Gain  Gain=ctrlConst.EncoderCountsPerRevolution/(2*pi)
      settings: AttributesFormatString=--------------------------------------------------\nGain:\n%<Gain>
  Discrete-Time Integrator : DiscreteIntegrator  InitialCondition=sensors.Encoder.InitialAngleRads  SampleTime=-1  ICPrevOutput=DiscIntNeverNeededParam  ICPrevScaledInput=DiscIntNeverNeededParam
      settings: AttributesFormatString=------------------------------\nInitial Condition: %<InitialCondition>
  Encoder Angle Data Type : DataTypeConversion  OutDataTypeStr=uint16  SaturateOnIntegerOverflow=off  RndMeth=Floor
  Math Function : Math  Operator=mod  SignedPower=on
  Radians Per Cycle : Constant  Value=2*pi
  Encoder Count : Outport  VectorParamsAs1DForOutWhenUnconnected=off
  wires:
  Radians Per Cycle/1 -> Math Function/2
  Math Function/1 -> Counts per Radian/1
  Counts per Radian/1 -> Encoder Angle Data Type/1
  Rotor Velocity/1 -> Discrete-Time Integrator/1
  Encoder Angle Data Type/1 -> Encoder Count/1
  Discrete-Time Integrator/1 -> Math Function/1

== system PMSMSystem/Embedded Processor/Sensor Peripherals/Measure Rotor Position (Quadrature Encoder)/Encoder Count (Valid After First Index Pulse) ==
  note: Encoder Count (Valid After First Index Pulse)
  note: Model the count value provided by the encoder when the absolute position is known.
      | The absolute position is known after reaching the first index pulse.
      | The pulse train generated by the encoder is not modeled.
  Rotor Angle : Inport
  Add : Sum
  Counts per Radian : Gain  Gain=ctrlConst.EncoderCountsPerRevolution/(2*pi)
      settings: AttributesFormatString=-------------------------------------------\nGain:\n%<Gain>
  Encoder Angle Data Type : DataTypeConversion  OutDataTypeStr=uint16  SaturateOnIntegerOverflow=off  RndMeth=Floor
  Math Function : Math  Operator=mod  SignedPower=on
  Offset_Between_Mechanical_Zero_And_Encoder_Zero : Constant  Value=sensors.Encoder.MechanicalToEncoderZeroOffsetRads
  Radians Per Cycle : Constant  Value=2*pi
  Encoder Count : Outport  VectorParamsAs1DForOutWhenUnconnected=off
  wires:
  Encoder Angle Data Type/1 -> Encoder Count/1
  Counts per Radian/1 -> Encoder Angle Data Type/1
  Radians Per Cycle/1 -> Math Function/2
  Offset_Between_Mechanical_Zero_And_Encoder_Zero/1 -> Add/2
  Math Function/1 -> Counts per Radian/1
  Rotor Angle/1 -> Add/1
  Add/1 -> Math Function/1

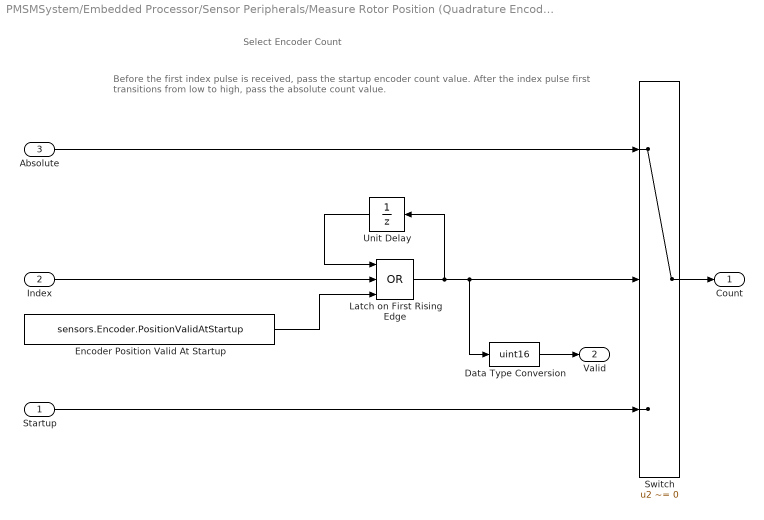
== system PMSMSystem/Embedded Processor/Sensor Peripherals/Measure Rotor Position (Quadrature Encoder)/Select Encoder Count ==
  note: Select Encoder Count
  note: Before the first index pulse is received, pass the startup encoder count value.
      | After the index pulse first transitions from low to high, pass the absolute count value.
  Startup : Inport
  Index : Inport  Port=2
  Absolute : Inport  Port=3
  Data Type Conversion : DataTypeConversion  OutDataTypeStr=uint16  SaturateOnIntegerOverflow=off  RndMeth=Floor
  Encoder Position Valid At Startup : Constant  Value=sensors.Encoder.PositionValidAtStartup
  Latch on First Rising Edge : Logic  Operator=OR  Inputs=3  IconShape=distinctive  AllPortsSameDT=off  OutDataTypeStr=boolean
  Switch : Switch  Criteria=u2 ~= 0  SaturateOnIntegerOverflow=off  InputSameDT=off
  Unit Delay : UnitDelay  SampleTime=-1  HasFrameUpgradeWarning=on
  Count : Outport  VectorParamsAs1DForOutWhenUnconnected=off
  Valid : Outport  Port=2  VectorParamsAs1DForOutWhenUnconnected=off
  wires:
  Latch on First Rising Edge/1 -> Unit Delay/1, Switch/2, Data Type Conversion/1
  Absolute/1 -> Switch/1
  Switch/1 -> Count/1
  Startup/1 -> Switch/3
  Unit Delay/1 -> Latch on First Rising Edge/1
  Index/1 -> Latch on First Rising Edge/2
  Encoder Position Valid At Startup/1 -> Latch on First Rising Edge/3
  Data Type Conversion/1 -> Valid/1

== matlab function PMSMSystem/Embedded Processor/Sensor Peripherals/Measure Rotor Position (Quadrature Encoder)/Create Index Pulse ==
  data: currentCount input; indexPulse output size=1; ctrlConst parameter
function indexPulse = fcn( currentCount, ctrlConst )  %#codegen
% Create an index pulse at position 2pi

    persistent previousCount;

    if isempty(previousCount)
        previousCount = currentCount;
    end

    % Detect the wrap. Assumes simulation will not allow moving pi rads
    % in one simulation step
    if abs(double(currentCount) - double(previousCount)) > (ctrlConst.EncoderCountsPerRevolution/2)
        index = true;
    else
        index = false;
    end

    previousCount = currentCount;

    indexPulse = uint16(index);
end
